simulink model "StepDownBalancedGrYGrY"  (R2023b)
settings: Solver=ode45  StartTime=0.0  StopTime=0.2  MaxStep=0.04  RelTol=1e-3
PreLoadFcn:
  | power_13NodeTestFeeder_init;
  | Ts=50e-6
undefined symbols (not defined in the file): C_4Bus, ft2km, L_4Bus, R_4Bus
libraries: spsLoadFlowBusLib x4, spsThreePhaseVIMeasurementLib x4, spsPiSectionLineLib x2, spsThreePhaseSeriesRLCLoadLib x1, spsThreePhaseSourceLib x1, spsThreePhaseTransformerTwoWindingsLib x1, spspowerguiLib x1
settings Model: Creator=The MathWorks, Inc.  LastModifiedBy=E1335542
settings SolverCC: AlgebraicLoopSolver=TrustRegion
settings DataIOCC: ExternalInput=getinputstruct(op_IEEE_13_node_5)  InitialState=getstatestruct(op_IEEE_13_node_5)  LimitDataPoints=on  SaveFormat=Array  ReturnWorkspaceOutputs=off
settings OptimizationCC: LifeSpan=inf
settings DebuggingCC: AlgebraicLoopMsg=none  FcnCallInpInsideContextMsg=warning  StateNameClashWarn=warning  SFUnexpectedBacktrackingDiag=warning  SFNoUnconditionalDefaultTransitionDiag=warning  SFExecutionAtInitializationDiag=none
settings ModelReferenceCC: EnableRefExpFcnMdlSchedulingChecks=on  PropagateSignalLabelsOutOfModel=off
settings SFSimCC: CustomCodeUndefinedFunction=UseInterfaceOnly
settings CodeAppCC: StateflowObjectComments=on
settings SimscapeCC: SimscapeNormalizeSystem=off

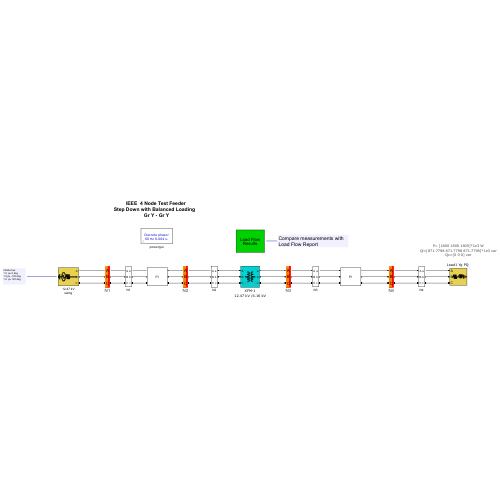
[thumbnail: Simulink's stored preview of the top-level diagram]
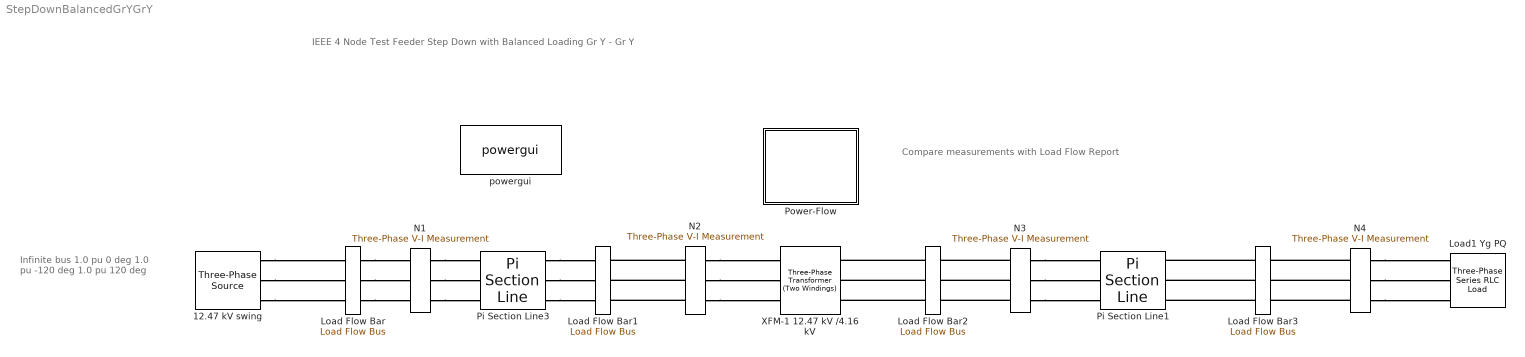
== system StepDownBalancedGrYGrY ==
  note: IEEE  4 Node Test Feeder
      | Step Down with Balanced Loading
      | Gr Y - Gr Y
  note: Compare measurements with
      | Load Flow Report
  note: Infinite bus
      | 1.0 pu 0 deg
      | 1.0 pu -120 deg
      | 1.0 pu 120 deg
  " Load1 Yg PQ " : spsThreePhaseSeriesRLCLoadLib/Three-Phase Series RLC Load  LConnTagsString=A|B|C  Configuration=Y (grounded)  NominalVoltage=120e3  Vabc=[ 0.799086 0.855098 0.8268]*2401.78  Vabcp=[1e3 1e3 1e3]  NominalFrequency=60  UnbalancedPower=on  ActivePower=1e+006  InductivePower=0  CapacitivePower=0  Pabc=[1800 1800 1800]*1e3  QLabc=[871.7798 871.7798 871.7798]*1e3  QCabc=[0 0 0]  Pabcp=[10e3 9e3 11e3]  QLabcp=[100 90 110]  QCabcp=[100 90 110]  Measurements=None  LoadType=constant PQ
      settings: AttributesFormatString=|
      | P= %<Pabc> W
      | Ql=%<QLabc> var
      | Qc=%<QCabc> var
  12.47 kV swing : spsThreePhaseSourceLib/Three-Phase Source  InternalConnection=Yg  VoltagePhases=on  Voltage=120e3  PhaseAngle=0  Voltage_phases=[ 1 1 1]*7199.56  PhaseAngles_phases=[ 0 -120 120]  Frequency=60  NonIdealSource=on  SpecifyImpedance=off  Resistance=1e-6  Inductance=0  ShortCircuitLevel=100e6  BaseVoltage=12.47e3  XRratio=10  BusType=swing  Pref=0  Qref=0  Prefabc=[0 0 0]  Qrefabc=[0 0 0]  Qmin="[-inf  -inf -inf]"  Qmax="[inf  inf inf]"
  Load Flow Bar : spsLoadFlowBusLib/Load Flow Bus  LConnTagsString=a|b|c  RConnTagsString=a|b|c  Phases=ABC  Connectors=on both sides  ID=N1  Vbase=12.47e3/sqrt(3)  Vref="[ 1.0  1.0  1.0]"  Vangle=[ 0 -120 120]  VLF=1  VLFb=1  VLFc=1  angleLF=0  angleLFb=-120  angleLFc=120
      settings: AttributesFormatString=%<ID>
  Load Flow Bar1 : spsLoadFlowBusLib/Load Flow Bus  LConnTagsString=a|b|c  RConnTagsString=a|b|c  Phases=ABC  Connectors=on both sides  ID=N2  Vbase=12.47e3/sqrt(3)  Vref=[1.0 1.0 1.0]  Vangle=[0 -120 120]  VLF=0.9877  VLFb=0.9908  VLFc=0.9892  angleLF=-0.2874  angleLFb=-120.4  angleLFc=119.6
      settings: AttributesFormatString=%<ID>
  Load Flow Bar2 : spsLoadFlowBusLib/Load Flow Bus  LConnTagsString=a|b|c  RConnTagsString=a|b|c  Phases=ABC  Connectors=on both sides  ID=N3  Vbase=4.16e3/sqrt(3)  Vref=[1.0 1.0 1.0]  Vangle=[0 -120 120]  VLF=0.9365  VLFb=0.9421  VLFc=0.9406  angleLF=-33.73  angleLFb=-153.4  angleLFc=86.36
      settings: AttributesFormatString=%<ID>
  Load Flow Bar3 : spsLoadFlowBusLib/Load Flow Bus  LConnTagsString=a|b|c  RConnTagsString=a|b|c  Phases=ABC  Connectors=on both sides  ID=N4  Vbase=4.16e3/sqrt(3)  Vref=[1.0 1.0 1.0]  Vangle=[0 -120 120]  VLF=0.7991  VLFb=0.8551  VLFc=0.8268  angleLF=-39.07  angleLFb=-158.3  angleLFc=80.85
      settings: AttributesFormatString=%<ID>
  N1 : spsThreePhaseVIMeasurementLib/Three-Phase V-I Measurement  VoltageMeasurement=phase-to-ground  SetLabelV=on  LabelV=Vabc_N1  Vpu=off  VpuLL=off  CurrentMeasurement=yes  SetLabelI=on  LabelI=Iabc_N1  Ipu=off  Pbase=100e6  Vbase=4160  OutputType=Complex  PhasorSimulation=on  PSBequivalent=0
  N2 : spsThreePhaseVIMeasurementLib/Three-Phase V-I Measurement  VoltageMeasurement=phase-to-ground  SetLabelV=on  LabelV=Vabc_N2  Vpu=off  VpuLL=off  CurrentMeasurement=yes  SetLabelI=on  LabelI=Iabc_N2  Ipu=off  Pbase=100e6  Vbase=4160  OutputType=Complex  PhasorSimulation=on  PSBequivalent=0
  N3 : spsThreePhaseVIMeasurementLib/Three-Phase V-I Measurement  VoltageMeasurement=phase-to-ground  SetLabelV=on  LabelV=Vabc_N3  Vpu=off  VpuLL=off  CurrentMeasurement=yes  SetLabelI=on  LabelI=Iabc_N3  Ipu=off  Pbase=100e6  Vbase=4160  OutputType=Complex  PhasorSimulation=on  PSBequivalent=0
  N4 : spsThreePhaseVIMeasurementLib/Three-Phase V-I Measurement  VoltageMeasurement=phase-to-ground  SetLabelV=on  LabelV=Vabc_N4  Vpu=off  VpuLL=off  CurrentMeasurement=yes  SetLabelI=on  LabelI=Iabc_N4  Ipu=off  Pbase=100e6  Vbase=4160  OutputType=Complex  PhasorSimulation=on  PSBequivalent=0
  Pi Section Line1 : spsPiSectionLineLib/Pi Section Line  LConnTagsString=1|i2|i3  RConnTagsString=1|o2|o3  Phases=3  PiSections=1  Length=2500*ft2km  Frequency=60  Resistance=R_4Bus  Inductance=L_4Bus  Capacitance=C_4Bus  SpecifyConductance=off  Conductance=0  Measurements=None  Measurements2=None
  Pi Section Line3 : spsPiSectionLineLib/Pi Section Line  LConnTagsString=1|i2|i3  RConnTagsString=1|o2|o3  Phases=3  PiSections=1  Length=2000*ft2km  Frequency=60  Resistance=R_4Bus  Inductance=L_4Bus  Capacitance=C_4Bus  SpecifyConductance=off  Conductance=0  Measurements=None  Measurements2=None
  Power-Flow : Subsystem
      mask Display: disp('Load Flow\nResults')
  XFM-1 12.47 kV /4.16 kV : spsThreePhaseTransformerTwoWindingsLib/Three-Phase Transformer (Two Windings)  Winding1Connection=Yg  Winding2Connection=Yg  CoreType=Three single-phase transformers  SetSaturation=off  Hysteresis=off  DataFile='hysteresis'  SetInitialFlux=off  Measurements=None  UNITS=pu  NominalPower=[ 6000e3 , 60 ]  Winding1=[12470 0.005 0.03]  Winding2=[4160 0.005 0.03]  Rm=500  Lm=500  L0=0.5  Saturation=[0 0;0.0024 1.2;1 1.52]  InitialFluxes=[0.8 -0.8 0.7]  BreakLoop=off  DiscreteSolver=Trapezoidal iterative  DataType=off  TransfoNumber=1
  powergui : spspowerguiLib/powergui  Priority=1  SimulationMode=Discrete phasor  SampleTime=4e-3  frequency=60  Iterations=50  frequencyindice=60  Pbase=100e3  ErrMax=0.0001  UnitsV=kV  UnitsW=kW  buscounter=0  FunctionMessages=off  echomessages=off  EnableUseOfTLC=off  CurrentSourceSwitches=off  DisableSnubberDevices=off  DisableRonSwitches=off  DisableVfSwitches=off  DisplayEquations=off  AutomaticDiscreteSolvers=off  SolverType=Tustin/Backward Euler (TBE)  Interpol=off  ExternalGateDelay=off  methode=off  Ts=0  x0status=blocks  SPID=off  SwTol=0  HookPort=off  NonlinearTolerance=1e-4  nMaxIteration=100  ContinueOnMaxIteration=off  RestoreLinks=warning  ResistiveCurrentMeasurement=off  Frange=[0:2:500]  Ylog=off  Xlog=on  ShowGrid=off  save=off  variable=ZData  structure=0  ZoomFFT=on  StartTime=0.0  cycles=1  DisplayStyle=1  fundamental=60  FreqAxis=off  MaxFrequency=1000  frequencyindicesteady=1  RmsSteady=1  display=off
  connections:
  Load Flow Bar3/LConn1 -- Pi Section Line1/RConn1
  N2/LConn2 -- Load Flow Bar1/RConn2
  12.47 kV swing/RConn1 -- Load Flow Bar/LConn1
  N3/RConn1 -- Pi Section Line1/LConn1
  N3/LConn2 -- Load Flow Bar2/RConn2
  N4/RConn3 -- " Load1 Yg PQ "/LConn3
  Pi Section Line3/RConn3 -- Load Flow Bar1/LConn3
  Pi Section Line3/RConn1 -- Load Flow Bar1/LConn1
  Load Flow Bar2/LConn2 -- XFM-1 12.47 kV /4.16 kV/RConn2
  N1/RConn1 -- Pi Section Line3/LConn1
  N2/RConn3 -- XFM-1 12.47 kV /4.16 kV/LConn3
  N1/RConn2 -- Pi Section Line3/LConn2
  N1/RConn3 -- Pi Section Line3/LConn3
  Load Flow Bar3/LConn2 -- Pi Section Line1/RConn2
  N2/LConn1 -- Load Flow Bar1/RConn1
  N2/LConn3 -- Load Flow Bar1/RConn3
  N4/LConn2 -- Load Flow Bar3/RConn2
  Load Flow Bar2/LConn1 -- XFM-1 12.47 kV /4.16 kV/RConn1
  Pi Section Line3/RConn2 -- Load Flow Bar1/LConn2
  N2/RConn1 -- XFM-1 12.47 kV /4.16 kV/LConn1
  Load Flow Bar/RConn2 -- N1/LConn2
  N4/LConn1 -- Load Flow Bar3/RConn1
  12.47 kV swing/RConn3 -- Load Flow Bar/LConn3
  N3/RConn2 -- Pi Section Line1/LConn2
  N4/RConn2 -- " Load1 Yg PQ "/LConn2
  12.47 kV swing/RConn2 -- Load Flow Bar/LConn2
  Load Flow Bar2/LConn3 -- XFM-1 12.47 kV /4.16 kV/RConn3
  Load Flow Bar/RConn1 -- N1/LConn1
  N3/LConn3 -- Load Flow Bar2/RConn3
  N4/RConn1 -- " Load1 Yg PQ "/LConn1
  Load Flow Bar3/LConn3 -- Pi Section Line1/RConn3
  N3/LConn1 -- Load Flow Bar2/RConn1
  N4/LConn3 -- Load Flow Bar3/RConn3
  N2/RConn2 -- XFM-1 12.47 kV /4.16 kV/LConn2
  N3/RConn3 -- Pi Section Line1/LConn3
  Load Flow Bar/RConn3 -- N1/LConn3

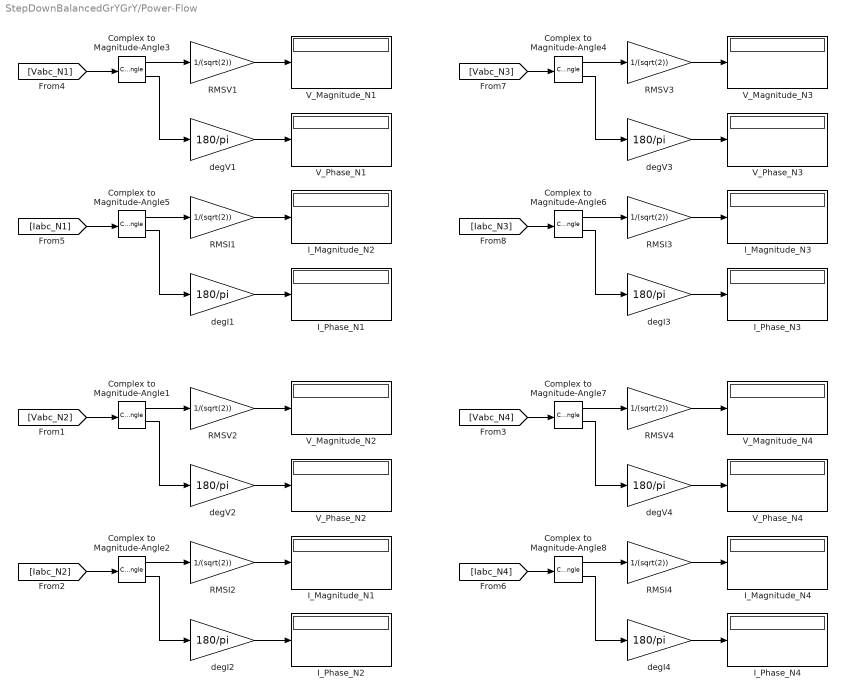
== system StepDownBalancedGrYGrY/Power-Flow ==
  Complex to Magnitude-Angle{1..8} (8 alike) : ComplexToMagnitudeAngle
  I_Magnitude_N{1..4} (4 alike) : Display
  I_Phase_N{1..4} (4 alike) : Display
  RMSI{1..4} (4 alike) : Gain  Gain=1/(sqrt(2))
  RMSV{1..4} (4 alike) : Gain  Gain=1/(sqrt(2))
  V_Magnitude_N{1..4} (4 alike) : Display
  V_Phase_N{1..4} (4 alike) : Display
  degI{1..4} (4 alike) : Gain  Gain=180/pi
  degV{1..4} (4 alike) : Gain  Gain=180/pi
  wires:
  RMSV1/1 -> V_Magnitude_N1/1
  [Vabc_N1] -> Complex to Magnitude-Angle3/1
  Complex to Magnitude-Angle3/1 -> RMSV1/1
  [Iabc_N1] -> Complex to Magnitude-Angle5/1
  degV1/1 -> V_Phase_N1/1
  Complex to Magnitude-Angle3/2 -> degV1/1
  degI1/1 -> I_Phase_N1/1
  Complex to Magnitude-Angle5/2 -> degI1/1
  Complex to Magnitude-Angle5/1 -> RMSI1/1
  RMSI1/1 -> I_Magnitude_N2/1
  RMSI2/1 -> I_Magnitude_N1/1
  degV2/1 -> V_Phase_N2/1
  Complex to Magnitude-Angle1/2 -> degV2/1
  [Iabc_N2] -> Complex to Magnitude-Angle2/1
  Complex to Magnitude-Angle1/1 -> RMSV2/1
  RMSV2/1 -> V_Magnitude_N2/1
  Complex to Magnitude-Angle2/1 -> RMSI2/1
  degI2/1 -> I_Phase_N2/1
  Complex to Magnitude-Angle2/2 -> degI2/1
  [Vabc_N2] -> Complex to Magnitude-Angle1/1
  RMSI3/1 -> I_Magnitude_N3/1
  degV3/1 -> V_Phase_N3/1
  Complex to Magnitude-Angle4/2 -> degV3/1
  [Iabc_N3] -> Complex to Magnitude-Angle6/1
  Complex to Magnitude-Angle4/1 -> RMSV3/1
  RMSV3/1 -> V_Magnitude_N3/1
  Complex to Magnitude-Angle6/1 -> RMSI3/1
  degI3/1 -> I_Phase_N3/1
  Complex to Magnitude-Angle6/2 -> degI3/1
  [Vabc_N3] -> Complex to Magnitude-Angle4/1
  Complex to Magnitude-Angle8/2 -> degI4/1
  Complex to Magnitude-Angle7/1 -> RMSV4/1
  degV4/1 -> V_Phase_N4/1
  Complex to Magnitude-Angle8/1 -> RMSI4/1
  degI4/1 -> I_Phase_N4/1
  RMSI4/1 -> I_Magnitude_N4/1
  RMSV4/1 -> V_Magnitude_N4/1
  Complex to Magnitude-Angle7/2 -> degV4/1
  [Iabc_N4] -> Complex to Magnitude-Angle8/1
  [Vabc_N4] -> Complex to Magnitude-Angle7/1
